simulink model "Body_ECU_SIL"  (R2026a)
settings: Solver=FixedStepAuto  StopTime=50  MaxStep=0.001  MinStep=0.0001  AbsTol=1e-6
InitFcn:
  | run('Vehicle_parameters_values_V1_MIL.m')
settings Model: PacingRate=0.500000  Creator=irfan  LastModifiedBy=irfan
settings SolverCC: ShapePreserveControl=EnableAll  ZeroCrossControl=EnableAll  ZeroCrossAlgorithm=Adaptive  MinimalZcImpactIntegration=on
settings DebuggingCC: ReadBeforeWriteMsg=DisableAll  WriteAfterWriteMsg=DisableAll  WriteAfterReadMsg=DisableAll  MultiTaskDSMMsg=none
settings SFSimCC: SFSimEcho=off
settings RTWCC: SystemTargetFile=ert.tlc  Description=Embedded Coder
settings ERTTargetCC: GenerateSampleERTMain=on  SupportContinuousTime=on

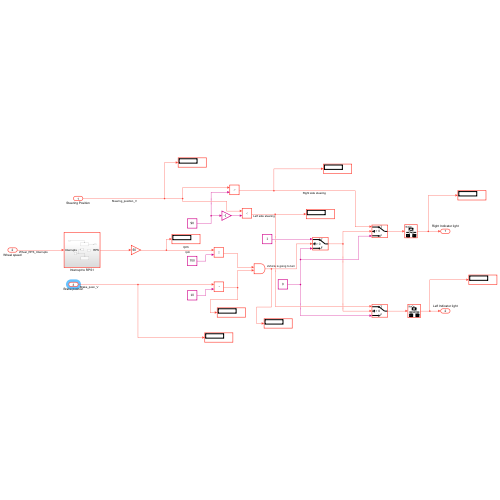
[thumbnail: Simulink's stored preview of the top-level diagram]
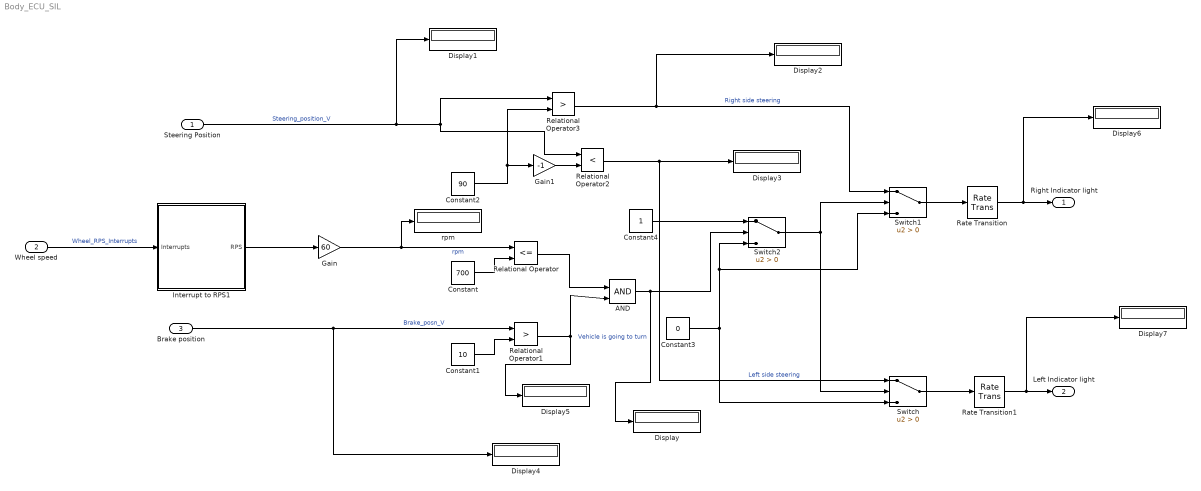
== system Body_ECU_SIL ==
  Steering Position : Inport  OutDataTypeStr=single  PortDimensions=1
  Wheel speed : Inport  Port=2  OutDataTypeStr=double  PortDimensions=1
  Brake position : Inport  Port=3  OutDataTypeStr=double  PortDimensions=1
  AND : Logic  IconShape=distinctive  AllPortsSameDT=off  OutDataTypeStr=boolean
  Constant : Constant  Value=700
  Constant1 : Constant  Value=10
  Constant2 : Constant  Value=90
  Constant3 : Constant  Value=0
  Constant4 : Constant
  Display{,1..7} (8 alike) : Display
  Gain : Gain  Gain=60
  Gain1 : Gain  Gain=-1
  Interrupt to RPS1 : Subsystem
  Rate Transition : RateTransition
  Rate Transition1 : RateTransition
  Relational Operator : RelationalOperator  Operator=<=  OutDataTypeStr=boolean  RndMeth=Simplest  InputSameDT=off
  Relational Operator1 : RelationalOperator  Operator=>  OutDataTypeStr=boolean  RndMeth=Simplest  InputSameDT=off
  Relational Operator2 : RelationalOperator  Operator=<  OutDataTypeStr=boolean  RndMeth=Simplest  InputSameDT=off
  Relational Operator3 : RelationalOperator  Operator=>  OutDataTypeStr=boolean  RndMeth=Simplest  InputSameDT=off
  Switch : Switch  Criteria=u2 > Threshold  SaturateOnIntegerOverflow=off  InputSameDT=off
  Switch1 : Switch  Criteria=u2 > Threshold  SaturateOnIntegerOverflow=off  InputSameDT=off
  Switch2 : Switch  Criteria=u2 > Threshold  SaturateOnIntegerOverflow=off  InputSameDT=off
  rpm : Display
  Right Indicator light : Outport  OutDataTypeStr=double  PortDimensions=1  SampleTime=[0,1]
  Left Indicator light : Outport  Port=2  OutDataTypeStr=double  PortDimensions=1  SampleTime=[0,1]
  wires:
  Rate Transition1/1 -> Left Indicator light/1, Display7/1
  Relational Operator/1 -> AND/1
  Rate Transition/1 -> Right Indicator light/1, Display6/1
  Constant1/1 -> Relational Operator1/2
  Constant4/1 -> Switch2/1
  Gain/1 -> rpm/1, Relational Operator/1  "rpm"
  Switch2/1 -> Switch1/2, Switch/2
  Constant/1 -> Relational Operator/2
  AND/1 -> Switch2/2, Display/1  "Vehicle is going to turn"
  Switch/1 -> Rate Transition1/1
  Constant2/1 -> Relational Operator3/2, Gain1/1
  Relational Operator1/1 -> Display5/1, AND/2
  Steering Position/1 -> Relational Operator2/1, Relational Operator3/1, Display1/1  "Steering_position_V"
  Brake position/1 -> Relational Operator1/1, Display4/1  "Brake_posn_V"
  Constant3/1 -> Switch2/3, Switch1/3, Switch/3
  Relational Operator2/1 -> Display3/1, Switch/1  "Left side steering"
  Relational Operator3/1 -> Switch1/1, Display2/1  "Right side steering"
  Switch1/1 -> Rate Transition/1
  Gain1/1 -> Relational Operator2/2
  Wheel speed/1 -> Interrupt to RPS1/1(Interrupts)  "Wheel_RPS_Interrupts"
  Interrupt to RPS1/1(RPS) -> Gain/1

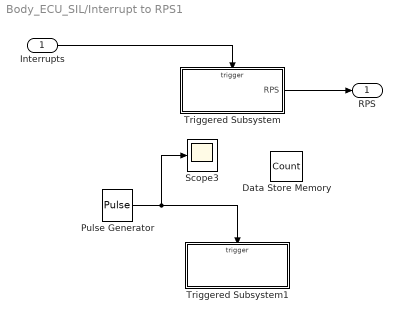
== system Body_ECU_SIL/Interrupt to RPS1 ==
  Interrupts : Inport
  Data Store Memory : DataStoreMemory  DataStoreName=Count  WriteAfterWriteMsg=warning  ShowAdditionalParam=off
  Pulse Generator : DiscretePulseGenerator  PulseType=Time based  Period=1.1  PulseWidth=10
  Scope3 : Scope
      settings: ActiveDisplayYMinimum=-0.12499999999999997  ActiveDisplayYMaximum=1.125  DataLoggingVariableName=ScopeData2
  Triggered Subsystem : Subsystem  TreatAsAtomicUnit=on
  Triggered Subsystem1 : Subsystem  TreatAsAtomicUnit=on
  RPS : Outport
  wires:
  Triggered Subsystem/1(RPS) -> RPS/1
  Pulse Generator/1 -> Triggered Subsystem1/Trigger, Scope3/1
  Interrupts/1 -> Triggered Subsystem/Trigger

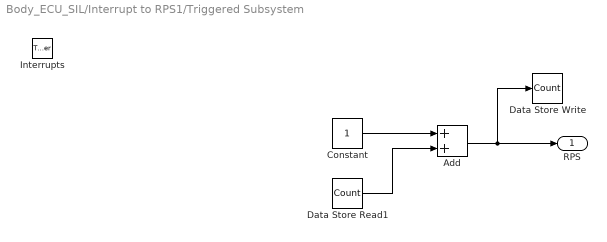
== system Body_ECU_SIL/Interrupt to RPS1/Triggered Subsystem ==
  Interrupts : TriggerPort  VariantControl=(inherit)
  Add : Sum
  Constant : Constant  SampleTime=-1
  Data Store Read1 : DataStoreRead  DataStoreName=Count  IndexOptions=Index vector (dialog)  Indices=1  OutputSizes=1
  Data Store Write : DataStoreWrite  DataStoreName=Count  IndexOptions=Index vector (dialog)  Indices=1  OutputSizes=1
  RPS : Outport
  wires:
  Data Store Read1/1 -> Add/2
  Add/1 -> RPS/1, Data Store Write/1
  Constant/1 -> Add/1

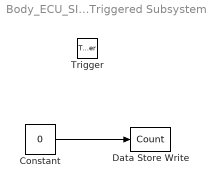
== system Body_ECU_SIL/Interrupt to RPS1/Triggered Subsystem1 ==
  Trigger : TriggerPort  VariantControl=(inherit)
  Constant : Constant  Value=0
  Data Store Write : DataStoreWrite  DataStoreName=Count  IndexOptions=Index vector (dialog)  Indices=1  OutputSizes=1
  wires:
  Constant/1 -> Data Store Write/1
